simulink model "sltestHeatpumpLibraryLinkExample"  (R2016a)
settings: Solver=FixedStepAuto  SolverMode=SingleTasking  StartTime=0.0  StopTime=30  FixedStep=.1  RelTol=1e-3
PostLoadFcn:
  | load 'sltestHeatpumpBusPostLoadFcn.mat'
  | load 'temp_input.mat'
model workspace (MAT data in the model file):
  Aw = Simulink.Parameter
  Aw.Value = 11.1540749554
  Aw.Description = 'Wall area, 12x10 ft'
  Aw.DataType = 'double'
  Aw.DocUnits = 'm^2'
  Aw.Dimensions = [1 1]
  Lw = Simulink.Parameter
  Lw.Value = 0.177800355601
  Lw.Description = '7 inch wall, expressed in meters'
  Lw.DataType = 'double'
  Lw.DocUnits = 'm'
  Lw.Dimensions = [1 1]
  V = Simulink.Parameter
  V.Value = 40.7932011331
  V.Description = 'Volume of the room (12x12x10ft) converted to m^3'
  V.DataType = 'double'
  V.DocUnits = 'm^3'
  V.Dimensions = [1 1]
  cpair = Simulink.Parameter
  cpair.Value = 1.004
  cpair.Description = 'specific heat of air, 1.004 kJ/kg-K'
  cpair.DataType = 'double'
  cpair.DocUnits = 'kJ/kg*K'
  cpair.Dimensions = [1 1]
  h = Simulink.Parameter
  h.Value = 25
  h.Description = 'Natural convection coefficient of heat transfer'
  h.DataType = 'double'
  h.DocUnits = 'W/m^2*K'
  h.Dimensions = [1 1]
  kw = Simulink.Parameter
  kw.Value = 0.67
  kw.Description = 'wall thermal conductivity, assuming a cinderblock wall'
  kw.DataType = 'double'
  kw.DocUnits = 'W/m*K'
  kw.Dimensions = [1 1]
  rhoair = Simulink.Parameter
  rhoair.Value = 1.22
  rhoair.Description = 'density of air'
  rhoair.DataType = 'double'
  rhoair.DocUnits = 'kg/m^3'
  rhoair.Dimensions = [1 1]
libraries: sltestHeatpumpLibraryExample x1
settings Model: Creator=The MathWorks, Inc.  LastModifiedBy=The MathWorks, Inc.
settings DataIOCC: ExternalInput=[t,u]  LimitDataPoints=on  SaveFormat=Array
settings DebuggingCC: SolverPrmCheckMsg=warning  AllowSymbolicDim=off
settings HardwareCC: ProdBitPerPointer=32  ProdLargestAtomicFloat=None  ProdIntDivRoundTo=Undefined  ProdEndianess=Unspecified  ProdWordSize=32  ProdHWDeviceType=32-bit Generic
settings ModelReferenceCC: PropagateSignalLabelsOutOfModel=off
settings ConfigComp: CovModelRefEnable=Off  CovSFcnEnable=off

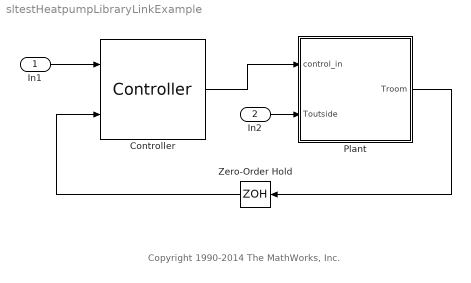
== system sltestHeatpumpLibraryLinkExample ==
  note: Copyright 1990-2014 The MathWorks, Inc.
  In1 : Inport
  In2 : Inport  Port=2
  Controller : sltestHeatpumpLibraryExample/Controller
  Plant : Subsystem  TreatAsAtomicUnit=on
      settings: MinAlgLoopOccurrences=on
  Zero-Order Hold : ZeroOrderHold
  wires:
  Controller/1 -> Plant/1(control_in)
  Plant/1(Troom) -> Zero-Order Hold/1
  Zero-Order Hold/1 -> Controller/2
  In2/1 -> Plant/2(Toutside)
  In1/1 -> Controller/1

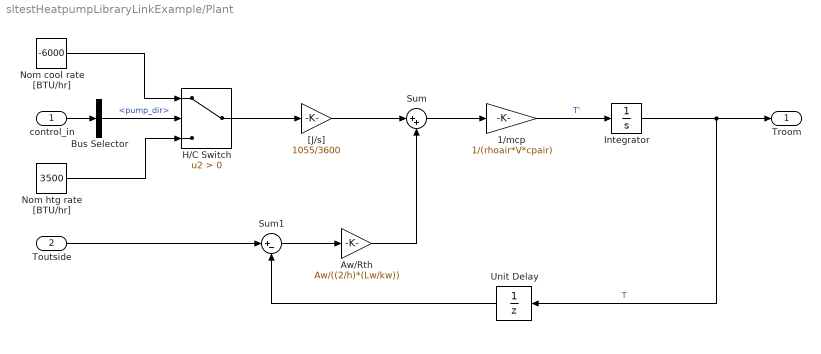
== system sltestHeatpumpLibraryLinkExample/Plant ==
  control_in : Inport
  Toutside : Inport  Port=2
  1/mcp : Gain  Gain=1/(rhoair*V*cpair)
  Aw/Rth : Gain  Gain=Aw/((2/h)*(Lw/kw))
  Bus Selector : BusSelector  OutputSignals=pump_dir
  H/C Switch : Switch  Criteria=u2 > Threshold
  Integrator : Integrator  InitialCondition=75
  Nom cool rate [BTU/hr] : Constant  Value=-6000
  Nom htg rate [BTU/hr] : Constant  Value=3500
  Sum : Sum  Inputs=|++
  Sum1 : Sum  Inputs=|+-
  Unit Delay : UnitDelay  InitialCondition=75  SampleTime=-1
  "[J/s]" : Gain  Gain=1055/3600
  Troom : Outport
  wires:
  Integrator/1 -> Unit Delay/1, Troom/1  "T"
  Bus Selector/1 -> H/C Switch/2  "<pump_dir>"
  control_in/1 -> Bus Selector/1
  Toutside/1 -> Sum1/1
  Nom cool rate [BTU/hr]/1 -> H/C Switch/1
  Nom htg rate [BTU/hr]/1 -> H/C Switch/3
  H/C Switch/1 -> "[J/s]"/1
  "[J/s]"/1 -> Sum/1
  Unit Delay/1 -> Sum1/2
  Sum1/1 -> Aw/Rth/1
  Aw/Rth/1 -> Sum/2
  1/mcp/1 -> Integrator/1  "T'"
  Sum/1 -> 1/mcp/1
